simulink model "SimNL"  (Simulink 7.6)
settings: Solver=ode45  StartTime=0.0  StopTime=100.0  RelTol=1e-3
values from neighbouring files (symbols this model uses):
  ParamReels =     [DataLin.mat]    (also in DataNLin.mat; LanceSimFK.m = ParamR)
settings Model: Creator=Mechbal  LastModifiedBy=Mechbal
settings OptimizationCC: BlockReduction=off  BooleanDataType=off
settings DebuggingCC: SaveWithParameterizedLinksMsg=none  SignalResolutionControl=TryResolveAllWithWarning  SolverPrmCheckMsg=none  MultiTaskDSMMsg=warning  MultiTaskCondExecSysMsg=none  StrictBusMsg=None
settings HardwareCC: TargetUnknown=on
settings RTWCC: IncludeERTFirstTime=on

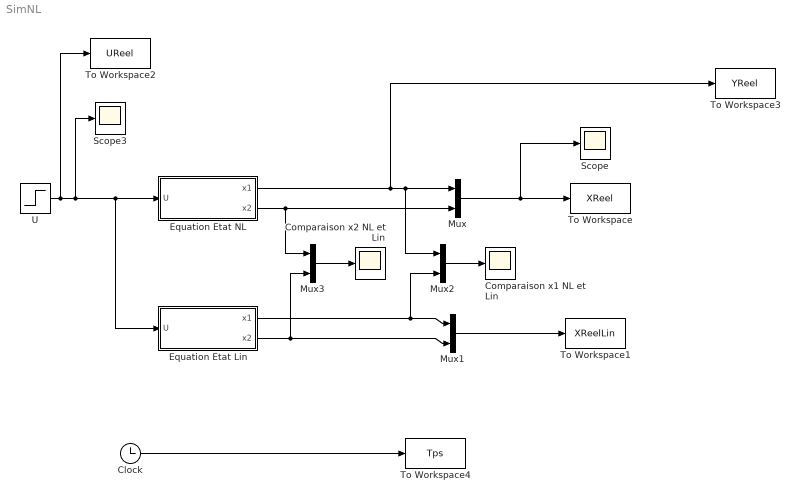
== system SimNL ==
  Clock : Clock
      settings: Decimation=10
  Comparaison x1 NL et Lin : Scope
  Comparaison x2 NL et Lin : Scope
      settings: SaveName=ScopeData2
  Equation Etat Lin : Subsystem
  Equation Etat NL : Subsystem
  Mux{,1..3} (4 alike) : Mux  Inputs=2
  Scope : Scope
  Scope3 : Scope
      settings: SaveName=ScopeData3
  To Workspace : ToWorkspace  VariableName=XReel  SampleTime=ParamReels.Te  SaveFormat=Array
  To Workspace1 : ToWorkspace  VariableName=XReelLin  SampleTime=ParamReels.Te  SaveFormat=Array
  To Workspace2 : ToWorkspace  VariableName=UReel  SampleTime=ParamReels.Te  SaveFormat=Array
  To Workspace3 : ToWorkspace  VariableName=YReel  SampleTime=ParamReels.Te  SaveFormat=Array
  To Workspace4 : ToWorkspace  VariableName=Tps  SampleTime=ParamReels.Te  SaveFormat=Array
  U : Step  Time=4  Before=ParamReels.Equilibre.Ue  After=ParamReels.Equilibre.Ue+1  SampleTime=0
  wires:
  U/1 -> Equation Etat NL/1(U), Equation Etat Lin/1(U), Scope3/1, To Workspace2/1
  Equation Etat NL/2(x2) -> Mux/2, Mux3/1
  Equation Etat NL/1(x1) -> To Workspace3/1, Mux/1, Mux2/1
  Mux/1 -> To Workspace/1, Scope/1
  Clock/1 -> To Workspace4/1
  Mux1/1 -> To Workspace1/1
  Equation Etat Lin/1(x1) -> Mux1/1, Mux2/2
  Equation Etat Lin/2(x2) -> Mux1/2, Mux3/2
  Mux2/1 -> Comparaison x1 NL et Lin/1
  Mux3/1 -> Comparaison x2 NL et Lin/1

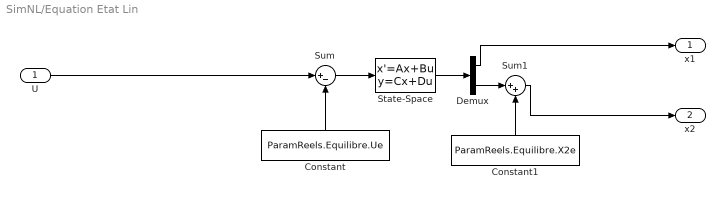
== system SimNL/Equation Etat Lin ==
  U : Inport
  Constant : Constant  Value=ParamReels.Equilibre.Ue
  Constant1 : Constant  Value=ParamReels.Equilibre.X2e
  Demux : Demux  Outputs=2
  State-Space : StateSpace  A=ParamReels.A  B=ParamReels.B  C=eye(2)  D=zeros(2,1)  X0=ParamReels.X0lin
  Sum : Sum  Inputs=|+-  SaturateOnIntegerOverflow=on  InputSameDT=on  OutDataTypeStr=Inherit: Same as first input
  Sum1 : Sum  Inputs=|++  SaturateOnIntegerOverflow=on  InputSameDT=on  OutDataTypeStr=Inherit: Same as first input
  x1 : Outport
  x2 : Outport  Port=2
  wires:
  State-Space/1 -> Demux/1
  U/1 -> Sum/1
  Sum/1 -> State-Space/1
  Constant/1 -> Sum/2
  Demux/2 -> Sum1/1
  Constant1/1 -> Sum1/2
  Sum1/1 -> x2/1
  Demux/1 -> x1/1

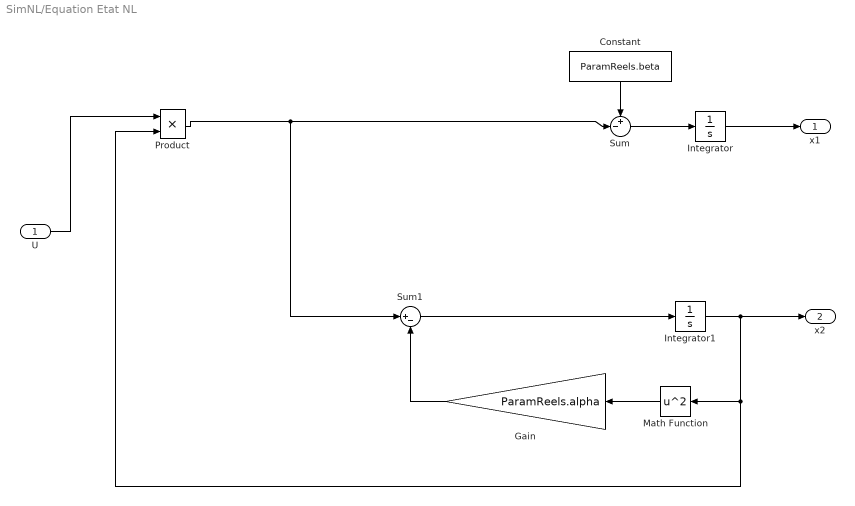
== system SimNL/Equation Etat NL ==
  U : Inport
  Constant : Constant  Value=ParamReels.beta
  Gain : Gain  Gain=ParamReels.alpha  SaturateOnIntegerOverflow=on  OutDataTypeStr=Inherit: Same as input  ParamDataTypeStr=Inherit: Same as input
  Integrator : Integrator  InitialCondition=ParamReels.X0(1,1)
  Integrator1 : Integrator  InitialCondition=ParamReels.X0(2,1)
  Math Function : Math  Operator=square  SaturateOnIntegerOverflow=on
  Product : Product  SaturateOnIntegerOverflow=on  RndMeth=Zero  InputSameDT=on  OutDataTypeStr=Inherit: Same as first input
  Sum : Sum  Inputs=+-|  SaturateOnIntegerOverflow=on  InputSameDT=on  OutDataTypeStr=Inherit: Same as first input
  Sum1 : Sum  Inputs=|+-  SaturateOnIntegerOverflow=on  InputSameDT=on  OutDataTypeStr=Inherit: Same as first input
  x1 : Outport
  x2 : Outport  Port=2
  wires:
  Integrator1/1 -> x2/1, Product/2, Math Function/1
  Integrator/1 -> x1/1
  Sum/1 -> Integrator/1
  Product/1 -> Sum/2, Sum1/1
  U/1 -> Product/1
  Constant/1 -> Sum/1
  Math Function/1 -> Gain/1
  Sum1/1 -> Integrator1/1
  Gain/1 -> Sum1/2
